simulink model "M2linear_linearcontrol"  (R2020b)
settings: Solver=VariableStepAuto  StartTime=0.0  StopTime=10  RelTol=1e-6
InitFcn:
  | clear;
  | load('datainit.mat');
  | set_param('M2linear_linearcontrol/Python2Sim','value','zeros(1,4)');
  | k = 40000
values from neighbouring files (symbols this model uses):
  commun = ones(node_in_len,2)    [M2Env_init.m]    (also in datainit.mat = [1  1; 1  1]; parameterinit.mat = [0 0 0 0 0 0 0 0 0 0 0 0 ... (16 elements, 8x2)]; parameterinit_initial.mat = [0 0 0 0 0 0 0 0 0 0 0 0 ... (16 elements, 8x2)])
  d = [100 100]    [datainit.mat]    (also in initAll.m = ESinit.Kdroop(1:node_in_len); parameterinit.mat)
  DataDelay = rand([node_in_len 2])*0.0    [M2Env_init.m]    (also in datainit.mat = [0  0; 0  0]; parameterinit.mat = [0 0 0 0 0 0 0 0 0 0 0 0 ... (16 elements, 8x2)]; parameterinit_initial.mat = [0 0 0 0 0 0 0 0 0 0 0 0 ... (16 elements, 8x2)])
  dis = Y(node_in,node_out)/(Y(node_out,node_out))*loadn    [M2Env_init.m]    (also in datainit.mat = [-6.36604493243 0])
  L = [14.2615268006  -14.2615268006; -14.2615268006  14.2615268006]    [datainit.mat]    (also in parameterinit.mat)
  m = [50 50]    [datainit.mat]    (also in initAll.m = ESinit.Kir(1:node_in_len); parameterinit.mat)
  wB = 314.159265359    [datainit.mat]    (also in parameterinit.mat; parameterinit_initial.mat)
libraries: powerlib_meascontrol x2
settings Model: Creator=Qiufan_Yang  LastModifiedBy=YangQiufan
settings SolverCC: AlgebraicLoopSolver=LineSearch
settings DataIOCC: DSMLogging=off  ReturnWorkspaceOutputs=off  SignalLoggingName=logout

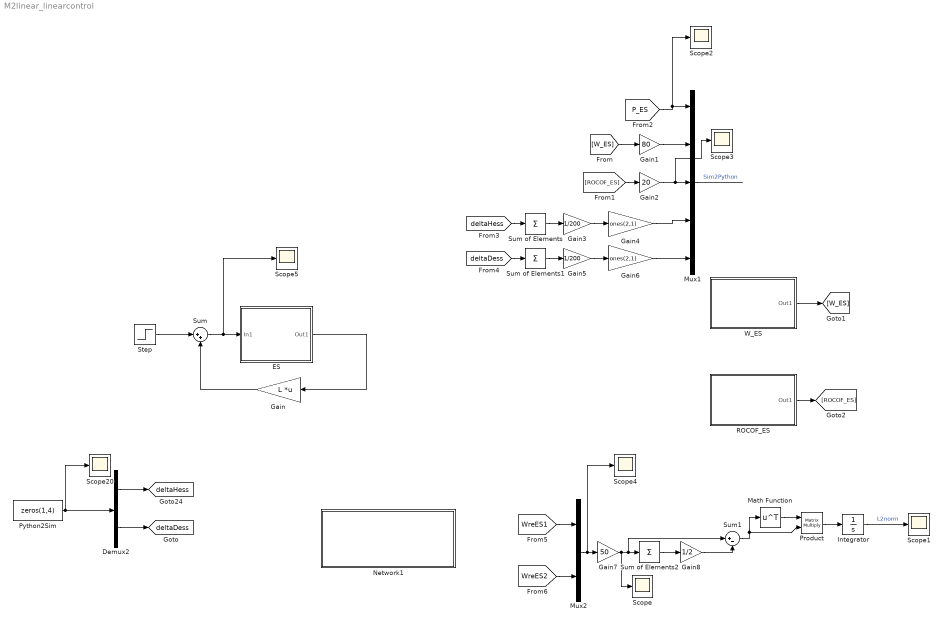
== system M2linear_linearcontrol ==
  Demux2 : Demux  Outputs=[2 2]
  ES : Subsystem
  Gain : Gain  Gain=L  Multiplication=Matrix(K*u)
  Gain1 : Gain  Gain=80
  Gain2 : Gain  Gain=20
  Gain3 : Gain  Gain=1/200
  Gain4 : Gain  Gain=ones(2,1)
  Gain5 : Gain  Gain=1/200
  Gain6 : Gain  Gain=ones(2,1)
  Gain7 : Gain  Gain=50
  Gain8 : Gain  Gain=1/2
  Integrator : Integrator
  Math Function : Math  Operator=transpose  SaturateOnIntegerOverflow=on
  Mux1 : Mux  Inputs=5
  Mux2 : Mux  Inputs=2
  Network1 : Subsystem
  Product : Product  Multiplication=Matrix(*)
  Python2Sim : Constant  Value=zeros(1,4)
  ROCOF_ES : Subsystem
  Scope{,1..5,20} (7 alike) : Scope
  Step : Step  Time=0.4  After=dis  SampleTime=0
  Sum : Sum  Inputs=|++
  Sum of Elements : Sum  Inputs=+
  Sum of Elements1 : Sum  Inputs=+
  Sum of Elements2 : Sum  Inputs=+
  Sum1 : Sum  Inputs=|+-
  W_ES : Subsystem
  tag scope: deltaDess=global, deltaHess=global
  wires:
  Step/1 -> Sum/1
  Gain/1 -> Sum/2
  ES/1(Out1) -> Gain/1
  Python2Sim/1 -> Scope20/1, Demux2/1
  Demux2/2 -> [deltaDess]
  Demux2/1 -> [deltaHess]
  W_ES/1(Out1) -> [W_ES]
  ROCOF_ES/1(Out1) -> [ROCOF_ES]
  [W_ES] -> Gain1/1
  [ROCOF_ES] -> Gain2/1
  [deltaHess] -> Sum of Elements/1
  Sum of Elements/1 -> Gain3/1
  Gain3/1 -> Gain4/1
  Gain4/1 -> Mux1/4
  Sum of Elements1/1 -> Gain5/1
  [deltaDess] -> Sum of Elements1/1
  Gain5/1 -> Gain6/1
  Gain6/1 -> Mux1/5
  [P_ES] -> Scope2/1, Mux1/1
  Gain1/1 -> Mux1/2
  Gain2/1 -> Scope3/1, Mux1/3
  Mux1/1 -> ?  "Sim2Python"
  [WreES2] -> Mux2/2
  [WreES1] -> Mux2/1
  Mux2/1 -> Scope4/1, Gain7/1
  Gain7/1 -> Scope/1, Sum1/1, Sum of Elements2/1
  Sum of Elements2/1 -> Gain8/1
  Gain8/1 -> Sum1/2
  Sum1/1 -> Product/2, Math Function/1
  Math Function/1 -> Product/1
  Product/1 -> Integrator/1
  Integrator/1 -> Scope1/1  "L2norm"
  Sum/1 -> Scope5/1, ES/1(In1)

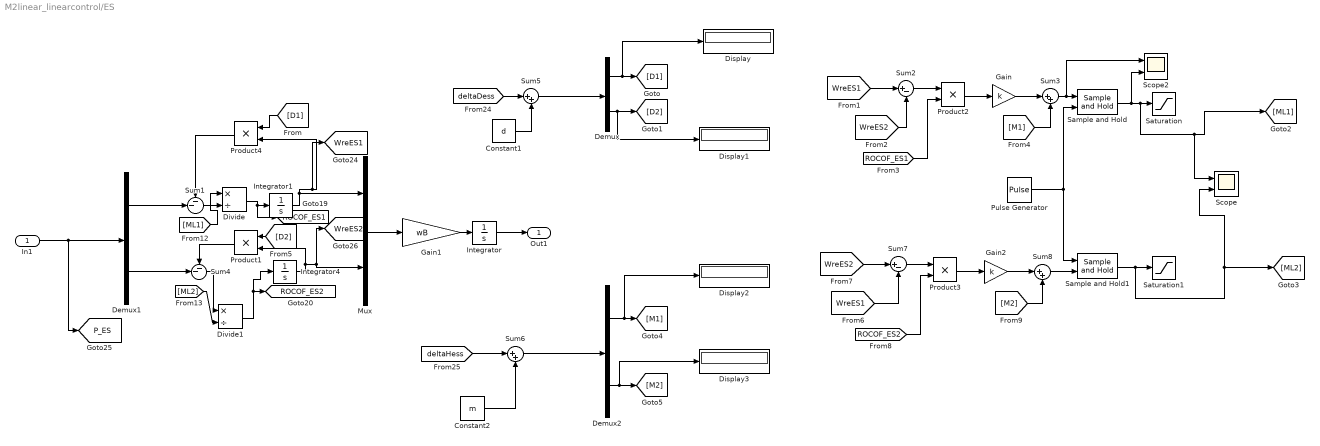
== system M2linear_linearcontrol/ES ==
  In1 : Inport
  Constant1 : Constant  Value=d
  Constant2 : Constant  Value=m
  Demux : Demux  Outputs=2
  Demux1 : Demux  Outputs=2
  Demux2 : Demux  Outputs=2
  Display{,1..3} (4 alike) : Display
  Divide : Product  Inputs=*/
  Divide1 : Product  Inputs=*/
  Gain : Gain  Gain=k
  Gain1 : Gain  Gain=wB  SaturateOnIntegerOverflow=on  OutDataTypeStr=Inherit: Same as input  ParamDataTypeStr=Inherit: Same as input
  Gain2 : Gain  Gain=k
  Integrator : Integrator
  Integrator1 : Integrator
  Integrator4 : Integrator
  Mux : Mux  Inputs=2
  Product{1..4} (4 alike) : Product
  Pulse Generator : DiscretePulseGenerator  PulseType=Time based  Period=0.2  PulseWidth=5
  Sample and Hold : powerlib_meascontrol/Additional Components/Sample and Hold  ic=0  Ts=0
      settings: SourceProductBaseCode=PS
  Sample and Hold1 : powerlib_meascontrol/Additional Components/Sample and Hold  ic=0  Ts=0
      settings: SourceProductBaseCode=PS
  Saturation : Saturate  UpperLimit=100  LowerLimit=0.1
  Saturation1 : Saturate  UpperLimit=100  LowerLimit=0.1
  Scope : Scope  NumInputPorts=2
  Scope2 : Scope  NumInputPorts=2
  Sum1 : Sum  Inputs=--|
  Sum2 : Sum  Inputs=|+-
  Sum{3,5..6,8} (4 alike) : Sum  Inputs=|++
  Sum4 : Sum  Inputs=--|
  Sum7 : Sum  Inputs=|+-
  Out1 : Outport
  tag scope: P_ES=global, ROCOF_ES1=global, ROCOF_ES2=global, WreES1=global, WreES2=global
  wires:
  Divide/1 -> [ROCOF_ES1], Integrator1/1
  Mux/1 -> Gain1/1
  Integrator4/1 -> Product1/2, Mux/2, [WreES2]
  In1/1 -> [P_ES], Demux1/1
  Product1/1 -> Sum4/1
  Product4/1 -> Sum1/1
  Integrator1/1 -> [WreES1], Product4/2, Mux/1
  Demux1/2 -> Sum4/2
  Demux1/1 -> Sum1/2
  Constant1/1 -> Sum5/2
  Demux/1 -> Display/1, [D1]
  Demux/2 -> Display1/1, [D2]
  [D1] -> Product4/1
  Constant2/1 -> Sum6/2
  Demux2/1 -> Display2/1, [M1]
  Demux2/2 -> Display3/1, [M2]
  [ML1] -> Divide/2
  [D2] -> Product1/1
  Sum4/1 -> Divide1/1
  Divide1/1 -> Integrator4/1, [ROCOF_ES2]
  [ML2] -> Divide1/2
  [deltaDess] -> Sum5/1
  [deltaHess] -> Sum6/1
  Gain1/1 -> Integrator/1
  Integrator/1 -> Out1/1
  Sum5/1 -> Demux/1
  Sum6/1 -> Demux2/1
  Sum1/1 -> Divide/1
  [WreES1] -> Sum2/1
  [WreES2] -> Sum2/2
  Sum2/1 -> Product2/1
  [ROCOF_ES1] -> Product2/2
  Product2/1 -> Gain/1
  Gain/1 -> Sum3/1
  [M1] -> Sum3/2
  Sample and Hold/1 -> Scope2/2, Scope/1, [ML1], Saturation/1
  Sum7/1 -> Product3/1
  Sample and Hold1/1 -> Scope/2, [ML2], Saturation1/1
  [M2] -> Sum8/2
  [ROCOF_ES2] -> Product3/2
  Product3/1 -> Gain2/1
  Sum8/1 -> Sample and Hold1/1
  Gain2/1 -> Sum8/1
  [WreES1] -> Sum7/2
  [WreES2] -> Sum7/1
  Pulse Generator/1 -> Sample and Hold/2, Sample and Hold1/2
  Sum3/1 -> Scope2/1, Sample and Hold/1

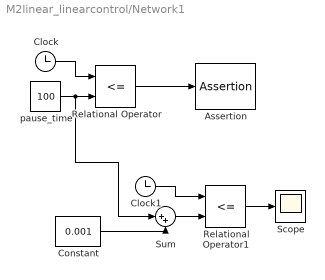
== system M2linear_linearcontrol/Network1 ==
  Assertion : Assertion  AssertionFailFcn=set_param(bdroot, 'SimulationCommand', 'pause');  StopWhenAssertionFail=off
  Clock : Clock
  Clock1 : Clock
  Constant : Constant  Value=0.001
  Relational Operator : RelationalOperator  Operator=<=  OutDataTypeStr=boolean  RndMeth=Simplest
  Relational Operator1 : RelationalOperator  Operator=<=  OutDataTypeStr=boolean  RndMeth=Simplest
  Scope : Scope
  Sum : Sum  Inputs=|++
  pause_time : Constant  Value=100
  wires:
  Relational Operator/1 -> Assertion/1
  Clock/1 -> Relational Operator/1
  pause_time/1 -> Sum/1, Relational Operator/2
  Sum/1 -> Relational Operator1/2
  Constant/1 -> Sum/2
  Clock1/1 -> Relational Operator1/1
  Relational Operator1/1 -> Scope/1

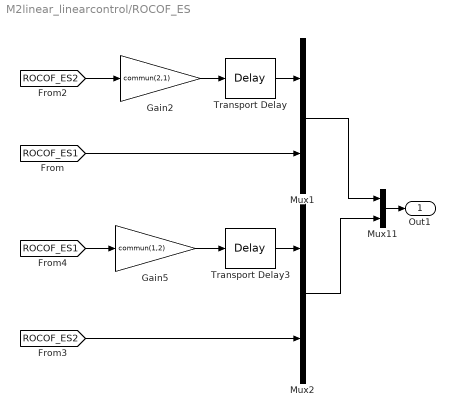
== system M2linear_linearcontrol/ROCOF_ES ==
  Gain2 : Gain  Gain=commun(2,1)
  Gain5 : Gain  Gain=commun(1,2)
  Mux1 : Mux  Inputs=2
  Mux11 : Mux  Inputs=2
  Mux2 : Mux  Inputs=2
  Transport Delay : TransportDelay  DelayTime=DataDelay(2,1)
  Transport Delay3 : TransportDelay  DelayTime=DataDelay(1,2)
  Out1 : Outport
  wires:
  Mux11/1 -> Out1/1
  Transport Delay3/1 -> Mux2/1
  Gain2/1 -> Transport Delay/1
  Mux2/1 -> Mux11/2
  [ROCOF_ES1] -> Gain5/1
  Mux1/1 -> Mux11/1
  [ROCOF_ES2] -> Gain2/1
  Gain5/1 -> Transport Delay3/1
  [ROCOF_ES2] -> Mux2/2
  [ROCOF_ES1] -> Mux1/2
  Transport Delay/1 -> Mux1/1

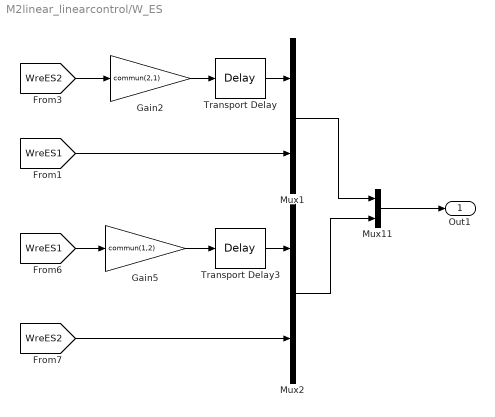
== system M2linear_linearcontrol/W_ES ==
  Gain2 : Gain  Gain=commun(2,1)
  Gain5 : Gain  Gain=commun(1,2)
  Mux1 : Mux  Inputs=2
  Mux11 : Mux  Inputs=2
  Mux2 : Mux  Inputs=2
  Transport Delay : TransportDelay  DelayTime=DataDelay(2,1)
  Transport Delay3 : TransportDelay  DelayTime=DataDelay(1,2)
  Out1 : Outport
  wires:
  [WreES2] -> Gain2/1
  Gain2/1 -> Transport Delay/1
  [WreES1] -> Gain5/1
  Gain5/1 -> Transport Delay3/1
  Transport Delay/1 -> Mux1/1
  [WreES2] -> Mux2/2
  Transport Delay3/1 -> Mux2/1
  [WreES1] -> Mux1/2
  Mux1/1 -> Mux11/1
  Mux2/1 -> Mux11/2
  Mux11/1 -> Out1/1
